simulink model "SwedishLighthousesHomework"  (R2016a)
settings: Solver=ode1  StartTime=0.0  StopTime=900  FixedStep=1  RelTol=1e-3
libraries: simulink x5, arduinolib x2
settings Model: ExtModeTrigDuration=2  Creator=dannen  LastModifiedBy=chris.barlow
settings DataIOCC: LimitDataPoints=on
settings OptimizationCC: OptimizeModelRefInitCode=on  LifeSpan=1  MaxStackSize=64
settings DebuggingCC: AllowSymbolicDim=off
settings HardwareCC: ProdBitPerInt=16  ProdBitPerPointer=16  ProdLargestAtomicFloat=None  ProdWordSize=8  ProdHWDeviceType=Atmel->AVR  UseEmbeddedCoderFeatures=off  UseSimulinkCoderFeatures=off
settings ModelReferenceCC: PropagateSignalLabelsOutOfModel=off
settings RTWCC: SystemTargetFile=ert.tlc  HardwareBoard=Arduino Uno  TemplateMakefile=ert_default_tmf  GenerateReport=on  Toolchain=Arduino AVR v1.6.1  BuildConfiguration=Faster Runs  IncludeHyperlinkInReport=on  LaunchReport=on  GenerateTraceInfo=on  GenerateTraceReport=on  GenerateTraceReportSl=on  GenerateTraceReportSf=on  GenerateTraceReportEml=on
settings CodeAppCC: ForceParamTrailComments=on  IgnoreCustomStorageClasses=off  OperatorAnnotations=on  SimulinkDataObjDesc=on  SFDataObjDesc=on  MATLABFcnDesc=on  InsertBlockDesc=on  MATLABSourceComments=on
settings ERTTargetCC: SupportContinuousTime=on  SupportNonInlinedSFcns=on  SupportVariableSizeSignals=on

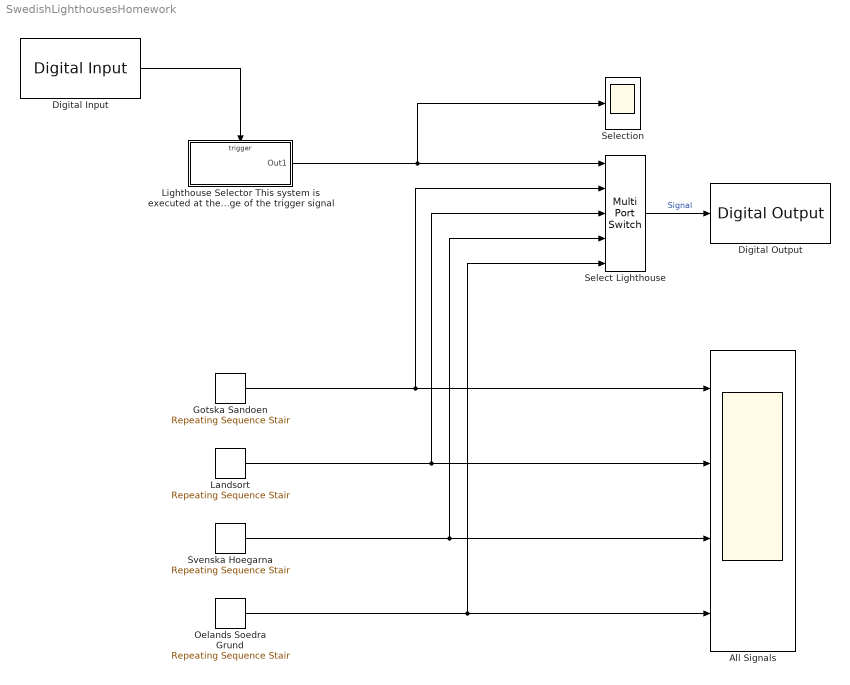
== system SwedishLighthousesHomework ==
  All Signals : Scope  NumInputPorts=4
  Digital Input : arduinolib/Digital Input  pinNumber=12  sampleTime=1  blockPlatform=arduino
  Digital Output : arduinolib/Digital Output  pinNumber=13  blockPlatform=arduino
  Gotska Sandoen : simulink/Sources/Repeating Sequence Stair  OutValues=[1 0 0 0 0]  tsamp=-1  OutMin=[]  OutMax=[]  OutDataTypeStr=double  OutputDataTypeScalingMode=double  OutDataType=fixdt(0,8)  ConRadixGroup=Best Precision: Vector-wise  OutScaling=2^-12
  Landsort : simulink/Sources/Repeating Sequence Stair  OutValues=[1 0 0 0 0 0 0 0 1 0 1 0 1 0 1 0 0 0 0 0 0 0 0 0 0 0 0 0 0 0 0 0 0 0 0 0 0 0 0 0 0 0 0 0 0 0 0 0 0 0 0 0 0 0 0 0 0 0 0 0 ]  tsamp=-1  OutMin=[]  OutMax=[]  OutDataTypeStr=double  OutputDataTypeScalingMode=double  OutDataType=fixdt(0,8)  ConRadixGroup=Best Precision: Vector-wise  OutScaling=2^-12
  Lighthouse Selector This system is executed at the rising edge of the trigger signal : Subsystem  TreatAsAtomicUnit=on
  Oelands Soedra Grund : simulink/Sources/Repeating Sequence Stair  OutValues=[ 1 1 1 1 0 0 0 0 ]  tsamp=-1  OutMin=[]  OutMax=[]  OutDataTypeStr=double  OutputDataTypeScalingMode=double  OutDataType=fixdt(0,8)  ConRadixGroup=Best Precision: Vector-wise  OutScaling=2^-12
  Select Lighthouse : MultiPortSwitch  Inputs=4  DiagnosticForDefault=None
  Selection : Scope
  Svenska Hoegarna : simulink/Sources/Repeating Sequence Stair  OutValues=[ 1 1 1 1 0 0 0 0 0 0 0 0 0 0 0 ]  tsamp=-1  OutMin=[]  OutMax=[]  OutDataTypeStr=double  OutputDataTypeScalingMode=double  OutDataType=fixdt(0,8)  ConRadixGroup=Best Precision: Vector-wise  OutScaling=2^-12
  wires:
  Gotska Sandoen/1 -> Select Lighthouse/2, All Signals/1
  Landsort/1 -> Select Lighthouse/3, All Signals/2
  Svenska Hoegarna/1 -> Select Lighthouse/4, All Signals/3
  Oelands Soedra Grund/1 -> Select Lighthouse/5, All Signals/4
  Lighthouse Selector This system is executed at the rising edge of the trigger signal/1(Out1) -> Select Lighthouse/1, Selection/1
  Digital Input/1 -> Lighthouse Selector This system is executed at the rising edge of the trigger signal/Trigger
  Select Lighthouse/1 -> Digital Output/1  "Signal"

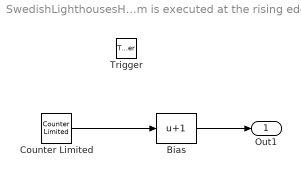
== system SwedishLighthousesHomework/Lighthouse Selector This system is executed at the rising edge of the trigger signal ==
  Trigger : TriggerPort  VariantControl=Variant
  Bias : Bias  Bias=1
  Counter Limited : simulink/Sources/Counter Limited  uplimit=3  tsamp=-1
  Out1 : Outport
  wires:
  Bias/1 -> Out1/1
  Counter Limited/1 -> Bias/1
